simulink model "shell"  (R2016b)
settings: Solver=VariableStepAuto  StartTime=0.0  StopTime=10.0  RelTol=1e-3
libraries: cstblocks x3
settings Model: Creator=m184410  LastModifiedBy=m181524

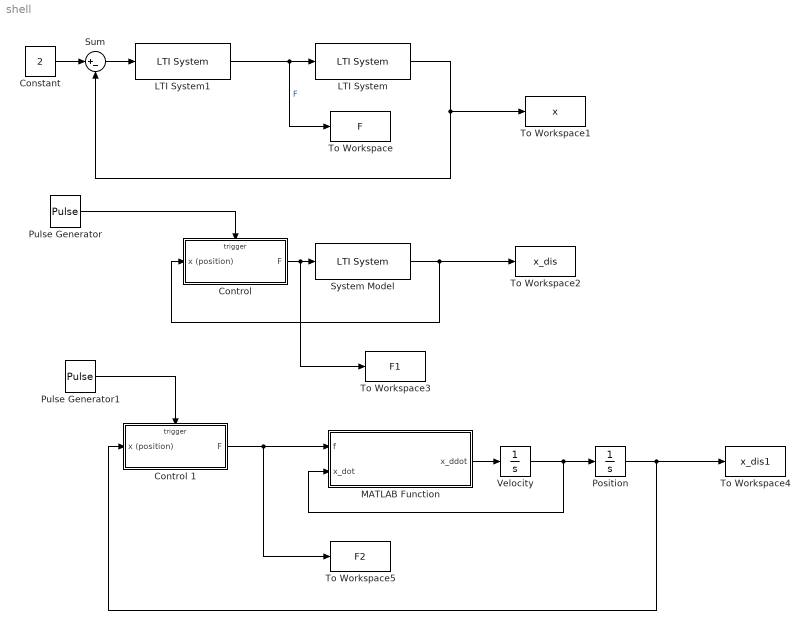
== system shell ==
  Constant : Constant  Value=2
  "Control " : Subsystem  TreatAsAtomicUnit=on
  Control 1 : Subsystem  TreatAsAtomicUnit=on
  LTI System : cstblocks/LTI System  sys=G  IC=[]
  LTI System1 : cstblocks/LTI System  sys=KGc  IC=[]
  MATLAB Function : MATLAB Function  TreatAsAtomicUnit=on
  Position : Integrator
  Pulse Generator : DiscretePulseGenerator  PulseType=Time based  Period=.01
  Pulse Generator1 : DiscretePulseGenerator  PulseType=Time based  Period=.01
  Sum : Sum  Inputs=|+-
  System Model : cstblocks/LTI System  sys=G  IC=[]
  To Workspace : ToWorkspace  VariableName=F  SaveFormat=Timeseries  SampleTime=-1
  To Workspace1 : ToWorkspace  VariableName=x  SaveFormat=Timeseries  SampleTime=-1
  To Workspace2 : ToWorkspace  VariableName=x_dis  SaveFormat=Timeseries  SampleTime=-1
  To Workspace3 : ToWorkspace  VariableName=F1  SaveFormat=Timeseries  SampleTime=-1
  To Workspace4 : ToWorkspace  VariableName=x_dis1  SaveFormat=Timeseries  SampleTime=-1
  To Workspace5 : ToWorkspace  VariableName=F2  SaveFormat=Timeseries  SampleTime=-1
  Velocity : Integrator
  wires:
  Sum/1 -> LTI System1/1
  LTI System1/1 -> To Workspace/1, LTI System/1  "F"
  Constant/1 -> Sum/1
  LTI System/1 -> To Workspace1/1, Sum/2
  "Control "/1("F ") -> To Workspace3/1, System Model/1
  System Model/1 -> To Workspace2/1, "Control "/1(x (position))
  Pulse Generator/1 -> "Control "/Trigger
  Control 1/1("F ") -> To Workspace5/1, MATLAB Function/1(f)
  Pulse Generator1/1 -> Control 1/Trigger
  MATLAB Function/1(x_ddot) -> Velocity/1
  Velocity/1 -> MATLAB Function/2(x_dot), Position/1
  Position/1 -> Control 1/1(x (position)), To Workspace4/1

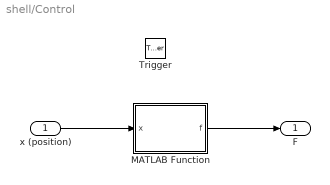
== system shell/Control  ==
  x (position) : Inport
  Trigger : TriggerPort  VariantControl=Variant
  MATLAB Function : MATLAB Function  TreatAsAtomicUnit=on
  "F " : Outport
  wires:
  x (position)/1 -> MATLAB Function/1(x)
  MATLAB Function/1(f) -> "F "/1

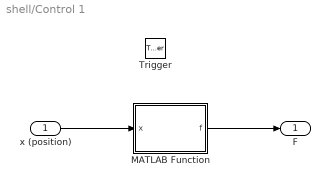
== system shell/Control 1 ==
  x (position) : Inport
  Trigger : TriggerPort  VariantControl=Variant
  MATLAB Function : MATLAB Function  TreatAsAtomicUnit=on
  "F " : Outport
  wires:
  x (position)/1 -> MATLAB Function/1(x)
  MATLAB Function/1(f) -> "F "/1

== matlab function shell/Control 1/MATLAB Function ==
  data: x input; f output
function f = es305_control(x)

persistent old_e old_f old2_e old2_f

if(isempty(old_e)) % checks to see if this is the first time running the func bc persistent creates an empty var if there was not previous value
        old_e=0.0;
        old_f=0.0;
        old2_e = 0.0;
        old2_f = 0.0;
end

x_ref=1.0; %desired position
e = x_ref - x; %x= actual position from sensor

f = 1.923076923076923*old_f -0.923076923076923*old2_f + 13.669296869657740*e -26.769269781977382*old_e + 13.107067708872410*old2_e;
% Age Vars
old2_e = old_e;
old2_f = old_f;
old_e=e;
old_f=f;

== matlab function shell/Control /MATLAB Function ==
  data: x input; f output
function f = es305_control(x)

persistent old_e old_f old2_e old2_f

if(isempty(old_e)) % checks to see if this is the first time running the func bc persistent creates an empty var if there was not previous value
        old_e=0.0;
        old_f=0.0;
        old2_e = 0.0;
        old2_f = 0.0;
end

x_ref=2.0; %desired position
e = x_ref - x; %x= actual position from sensor

f = 1.923076923076923*old_f -0.923076923076923*old2_f + 13.669296869657740*e -26.769269781977382*old_e + 13.107067708872410*old2_e;
% Age Vars
old2_e = old_e;
old2_f = old_f;
old_e=e;
old_f=f;
end

== matlab function shell/MATLAB Function ==
  data: f input; x_ddot output; x_dot input
function x_ddot = nonlinear_model(f,x_dot)

m = 1.0;
b = 0.1;
g = 9.81;

x_ddot = 1/m*(-b*x_dot+f+m*g);

end
